simulink model "CAT797_ADRC"  (R2026a)
settings: Solver=ode4  StopTime=30  FixedStep=0.0001
PreLoadFcn:
  | addpath("G:\Control_Research\Autonomy_Mining_Dump_Truck\src\plant_model\lib")
undefined symbols (not defined in the file): b1, b2, b3, Cf, Kd, Kp, Machine_Mass, Ts
libraries: simulink_extras x1, lat_dyn_haul_00 x1
settings Model: DataDictionary=CAT_797F.sldd  Creator=marti343  LastModifiedBy=Yahoff
settings OptimizationCC: EnableMemcpy=off
settings HardwareCC: ProdBitPerChar=16.0  ProdBitPerInt=16.0  ProdLargestAtomicInteger=Integer  ProdWordSize=16.0  ProdHWDeviceType=Texas Instruments->C2000
settings RTWCC: GenerateReport=on  LaunchReport=on
settings CodeAppCC: MATLABSourceComments=on

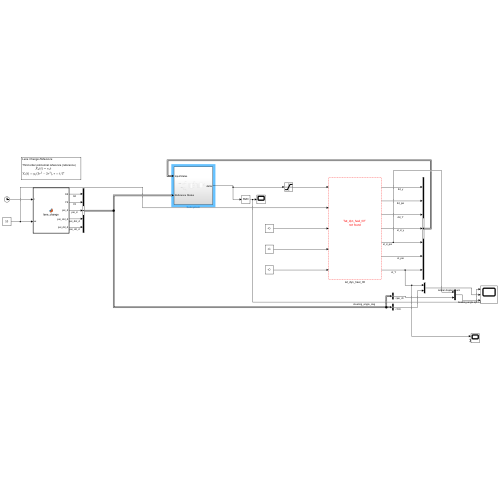
[thumbnail: Simulink's stored preview of the top-level diagram]
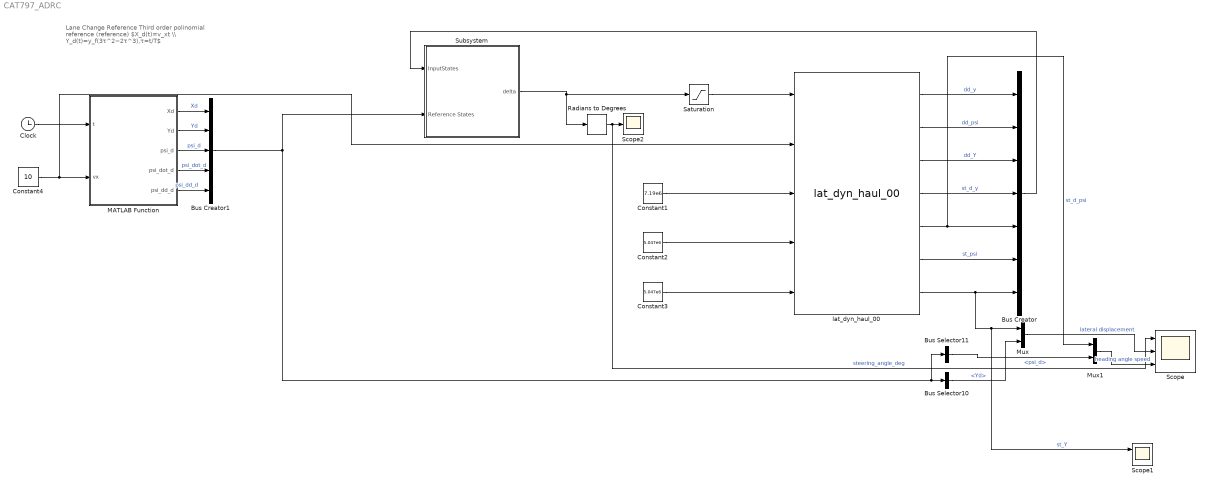
== system CAT797_ADRC ==
  note: Lane Change Reference
      |
      | Third order polinomial reference (reference)
      | $X_d​(t)=v_x​t \\ Y_d(t)=y_f(3τ^2−2τ^3),τ=t/T$
  Bus Creator : BusCreator  Inputs=7
  Bus Creator1 : BusCreator  Inputs=5
  Bus Selector10 : BusSelector  OutputSignals=Yd
  Bus Selector11 : BusSelector  OutputSignals=psi_d
  Clock : Clock
  Constant1 : Constant  Value=7.19e6
  Constant2 : Constant  Value=5.047e6
  Constant3 : Constant  Value=5.047e6
  Constant4 : Constant  Value=10
  MATLAB Function : MATLAB Function  TreatAsAtomicUnit=on
  Mux : Mux  Inputs=2
  Mux1 : Mux  Inputs=2
  Radians to Degrees : simulink_extras/Transformations/Radians to Degrees
  Saturation : Saturate  UpperLimit=25  LowerLimit=-25
  Scope : Scope  NumInputPorts=3
      settings: ActiveDisplayYMinimum=-0.88566383447217623  ActiveDisplayYMaximum=1.8819829612077903
  Scope1 : Scope  NumInputPorts=2
      settings: ActiveDisplayYMinimum=-3.5690828148427576  ActiveDisplayYMaximum=32.11098492285906
  Scope2 : Scope
      settings: ActiveDisplayYMinimum=-0.51210821519583338  ActiveDisplayYMaximum=1.8404657922652068  DataLoggingVariableName=ScopeData2
  Subsystem : Subsystem
  lat_dyn_haul_00 : lat_dyn_haul_00/lat_dyn_haul_00  SystemSampleTime=-1  SSRTWFcnClass=[]  VariantActivationTime=update diagram  EmptyChoice=off  PassThrough=off  PassThroughVariantControl=(default)  EmptyChoiceVariantControl=(default)  AllowFlexibleInterface=on  Latency=0  AutoFrameSizeCalculation=off
  wires:
  lat_dyn_haul_00/1 -> Bus Creator/1  "dd_y"
  lat_dyn_haul_00/3 -> Bus Creator/3  "dd_Y"
  lat_dyn_haul_00/4 -> Bus Creator/4  "st_d_y"
  Constant4/1 -> lat_dyn_haul_00/2, MATLAB Function/2(vx)
  Constant1/1 -> lat_dyn_haul_00/3
  Constant2/1 -> lat_dyn_haul_00/4
  Constant3/1 -> lat_dyn_haul_00/5
  Saturation/1 -> lat_dyn_haul_00/1
  lat_dyn_haul_00/2 -> Bus Creator/2  "dd_psi"
  lat_dyn_haul_00/6 -> Bus Creator/6  "st_psi"
  lat_dyn_haul_00/7 -> Scope1/1, Mux/1, Bus Creator/7  "st_Y"
  Clock/1 -> MATLAB Function/1(t)
  MATLAB Function/1(Xd) -> Bus Creator1/1  "Xd"
  MATLAB Function/2(Yd) -> Bus Creator1/2  "Yd"
  MATLAB Function/3(psi_d) -> Bus Creator1/3  "psi_d"
  MATLAB Function/4(psi_dot_d) -> Bus Creator1/4  "psi_dot_d"
  MATLAB Function/5(psi_dd_d) -> Bus Creator1/5  "psi_dd_d"
  Bus Creator1/1 -> Subsystem/2(Reference States), Bus Selector11/1, Bus Selector10/1
  Bus Selector10/1 -> Mux/2  "<Yd>"
  Bus Selector11/1 -> Mux1/2  "<psi_d>"
  lat_dyn_haul_00/5 -> Mux1/1, Bus Creator/5  "st_d_psi"
  Bus Creator/1 -> Subsystem/1(InputStates)
  Radians to Degrees/1 -> Scope/1, Scope2/1  "steering_angle_deg"
  Mux/1 -> Scope/2  "lateral displacement"
  Mux1/1 -> Scope/3  "heading angle speed"
  Subsystem/1(delta) -> Radians to Degrees/1, Saturation/1

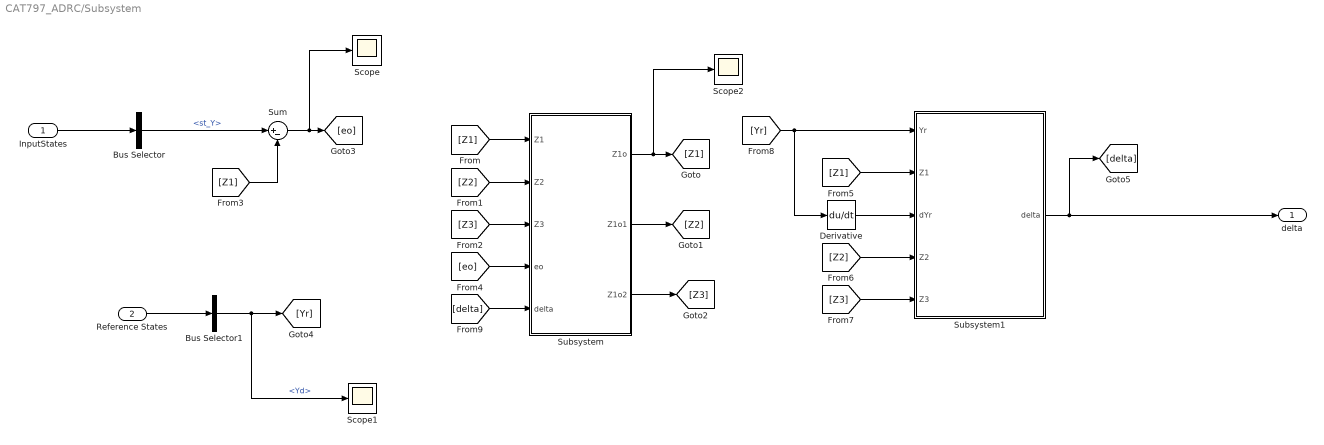
== system CAT797_ADRC/Subsystem ==
  InputStates : Inport
  Reference States : Inport  Port=2
  Bus Selector : BusSelector  OutputSignals=st_Y
  Bus Selector1 : BusSelector  OutputSignals=Yd
  Derivative : Derivative
  Scope : Scope
      settings: ActiveDisplayYMinimum=-0.00090570814196684667  ActiveDisplayYMaximum=0.00051399319976981963  DataLoggingVariableName=ScopeData3
  Scope1 : Scope
      settings: ActiveDisplayYMinimum=-0.43749999999999989  ActiveDisplayYMaximum=3.9375  DataLoggingVariableName=ScopeData4
  Scope2 : Scope
      settings: ActiveDisplayYMinimum=-1  ActiveDisplayYMaximum=1  DataLoggingVariableName=ScopeData5
  Subsystem : Subsystem
  Subsystem1 : Subsystem
  Sum : Sum  Inputs=|+-
  delta : Outport
  wires:
  InputStates/1 -> Bus Selector/1
  Subsystem/1(Z1o) -> Scope2/1, [Z1]
  Subsystem/2(Z1o1) -> [Z2]
  Subsystem/3(Z1o2) -> [Z3]
  [Z1] -> Subsystem/1(Z1)
  [Z2] -> Subsystem/2(Z2)
  [Z3] -> Subsystem/3(Z3)
  Bus Selector/1 -> Sum/1  "<st_Y>"
  [Z1] -> Sum/2
  Sum/1 -> Scope/1, [eo]
  [eo] -> Subsystem/4(eo)
  [delta] -> Subsystem/5(delta)
  [Z3] -> Subsystem1/5(Z3)
  [Z2] -> Subsystem1/4(Z2)
  [Z1] -> Subsystem1/2(Z1)
  Reference States/1 -> Bus Selector1/1
  Bus Selector1/1 -> Scope1/1, [Yr]  "<Yd>"
  [Yr] -> Derivative/1, Subsystem1/1(Yr)
  Derivative/1 -> Subsystem1/3(dYr)
  Subsystem1/1(delta) -> delta/1, [delta]

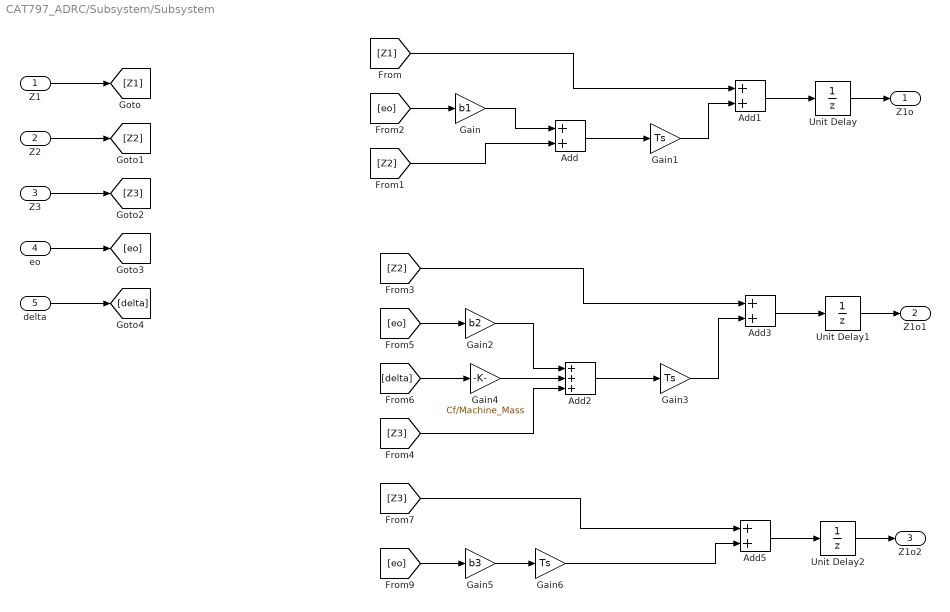
== system CAT797_ADRC/Subsystem/Subsystem ==
  Z1 : Inport
  Z2 : Inport  Port=2
  Z3 : Inport  Port=3
  eo : Inport  Port=4
  delta : Inport  Port=5
  Add{,1,3,5} (4 alike) : Sum
  Add2 : Sum  Inputs=+++
  Gain : Gain  Gain=b1
  Gain1 : Gain  Gain=Ts
  Gain2 : Gain  Gain=b2
  Gain3 : Gain  Gain=Ts
  Gain4 : Gain  Gain=Cf/Machine_Mass
  Gain5 : Gain  Gain=b3
  Gain6 : Gain  Gain=Ts
  Unit Delay : UnitDelay  SampleTime=-1
  Unit Delay1 : UnitDelay  SampleTime=-1
  Unit Delay2 : UnitDelay  SampleTime=-1
  Z1o : Outport
  Z1o1 : Outport  Port=2
  Z1o2 : Outport  Port=3
  wires:
  Z1/1 -> [Z1]
  Z2/1 -> [Z2]
  Z3/1 -> [Z3]
  eo/1 -> [eo]
  [eo] -> Gain/1
  Gain/1 -> Add/1
  [Z2] -> Add/2
  Add/1 -> Gain1/1
  [Z1] -> Add1/1
  Gain1/1 -> Add1/2
  Add1/1 -> Unit Delay/1
  Unit Delay/1 -> Z1o/1
  Gain3/1 -> Add3/2
  [eo] -> Gain2/1
  [Z2] -> Add3/1
  Unit Delay1/1 -> Z1o1/1
  [Z3] -> Add2/3
  Gain2/1 -> Add2/1
  Add3/1 -> Unit Delay1/1
  Add2/1 -> Gain3/1
  [delta] -> Gain4/1
  Gain4/1 -> Add2/2
  [eo] -> Gain5/1
  Add5/1 -> Unit Delay2/1
  Gain6/1 -> Add5/2
  Gain5/1 -> Gain6/1
  [Z3] -> Add5/1
  Unit Delay2/1 -> Z1o2/1
  delta/1 -> [delta]

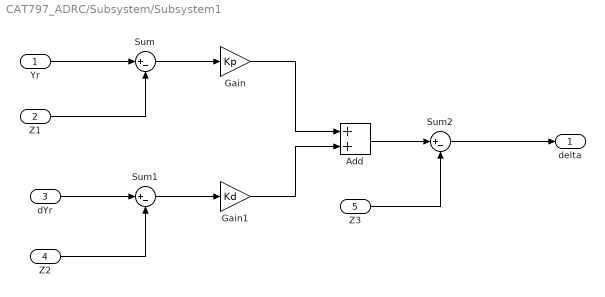
== system CAT797_ADRC/Subsystem/Subsystem1 ==
  Yr : Inport
  Z1 : Inport  Port=2
  dYr : Inport  Port=3
  Z2 : Inport  Port=4
  Z3 : Inport  Port=5
  Add : Sum
  Gain : Gain  Gain=Kp
  Gain1 : Gain  Gain=Kd
  Sum : Sum  Inputs=|+-
  Sum1 : Sum  Inputs=|+-
  Sum2 : Sum  Inputs=|+-
  delta : Outport
  wires:
  Yr/1 -> Sum/1
  Z1/1 -> Sum/2
  dYr/1 -> Sum1/1
  Z2/1 -> Sum1/2
  Sum/1 -> Gain/1
  Sum1/1 -> Gain1/1
  Gain/1 -> Add/1
  Gain1/1 -> Add/2
  Add/1 -> Sum2/1
  Z3/1 -> Sum2/2
  Sum2/1 -> delta/1

== matlab function CAT797_ADRC/MATLAB Function ==
  data: t input; Xd output; vx input; Yd output; psi_d output; psi_dot_d output; psi_dd_d output
function [Xd, Yd, psi_d, psi_dot_d, psi_dd_d] = lane_change(t, vx)

% PARAMETERS (tune these)
T  = 10;       % duration [s]
yf = 3.5;      % lateral shift [m]

% Normalize time
tau = t / T;

% Clamp tau between 0 and 1
if tau > 1
    tau = 1;
end
if tau < 0
    tau = 0;
end

% =========================
% POSITION
% =========================
Xd = vx * t;
Yd = yf * (3*tau^2 - 2*tau^3);

% =========================
% FIRST DERIVATIVE
% =========================
Xd_dot = vx;
Yd_dot = yf * (6*tau/T - 6*tau^2/T);

% =========================
% SECOND DERIVATIVE
% =========================
Xd_ddot = 0;
Yd_ddot = yf * (6/T^2 - 12*tau/T^2);

% =========================
% HEADING
% =========================
psi_d = atan2(Yd_dot, Xd_dot);

% =========================
% YAW RATE
% =========================
psi_dot_d = (Xd_dot * Yd_ddot - Yd_dot * Xd_ddot) / ...
            (Xd_dot^2 + Yd_dot^2);

% =========================
% YAW ACCELERATION (optional)
% =========================
% Numerical approximation (simple)
dt = 1e-3;

tau2 = (t+dt)/T;
if tau2 > 1
    tau2 = 1;
end

Yd_dot_2 = yf * (6*tau2/T - 6*tau2^2/T);
psi_d_2 = atan2(Yd_dot_2, vx);

psi_dd_d = (psi_d_2 - psi_d) / dt;

end
